simulink model "scExampleAutomotiveElectricalSystemAnalysis"  (R2024a)
settings: Solver=VariableStepAuto  StartTime=0.0  StopTime=10.0  RelTol=1e-3
(part 2 of 2)

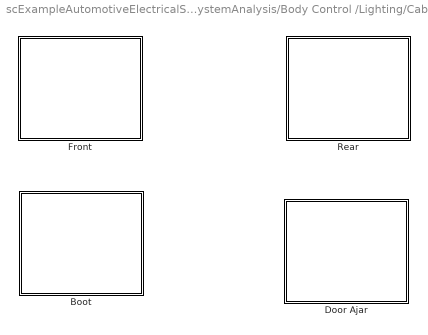
== system scExampleAutomotiveElectricalSystemAnalysis/Body Control /Lighting/Cabin lights ==
  Boot : Subsystem
      settings: PortSchema="{\"entries\":[{\"content\":{\"headerSize\":26,\"margin\":15,\"minimumSpacing\":25,\"sides\":[{\"content\":{\"connectorIds\":[]},\"type\":\"ConnectorPlacement.EquallySpacedRectSide\",\"uuid\":\"3d65bb45-329f-4bcb-b2ca-42a1dcaed35c\"},{\"content\":{\"connectorIds\":[],\"side\":\"RIGHT\"},\"type\":\"ConnectorPlacement.EquallySpacedRectSide\",\"uuid\":\"712ce926-4e36-4f57-ab01-804e3d1e4b50\"},{\"content\":{\"connectorIds\":[],\"side\":\"TOP\"},\"type\":\"ConnectorPlacement.EquallySpacedRectSide\",\"uuid\":\"e185dea3-2ee8-4adb-8a1b-2283728bdd8a\"}]},\"type\":\"ConnectorPlacement.EquallySpacedConnector\",\"uuid\":\"16f1484a-02ca-4d23-9e19-71fd982c775e\"}],\"packageUris\":[\"http:\\/\\/schema.mathworks.com\\/mf0\\/Connector\\/19700101\"],\"version\":\"1.0\"}"
  Door Ajar : Subsystem
      settings: PortSchema="{\"entries\":[{\"content\":{\"headerSize\":26,\"margin\":15,\"minimumSpacing\":25,\"sides\":[{\"content\":{\"connectorIds\":[]},\"type\":\"ConnectorPlacement.EquallySpacedRectSide\",\"uuid\":\"3d65bb45-329f-4bcb-b2ca-42a1dcaed35c\"},{\"content\":{\"connectorIds\":[],\"side\":\"RIGHT\"},\"type\":\"ConnectorPlacement.EquallySpacedRectSide\",\"uuid\":\"712ce926-4e36-4f57-ab01-804e3d1e4b50\"},{\"content\":{\"connectorIds\":[],\"side\":\"TOP\"},\"type\":\"ConnectorPlacement.EquallySpacedRectSide\",\"uuid\":\"e185dea3-2ee8-4adb-8a1b-2283728bdd8a\"}]},\"type\":\"ConnectorPlacement.EquallySpacedConnector\",\"uuid\":\"16f1484a-02ca-4d23-9e19-71fd982c775e\"}],\"packageUris\":[\"http:\\/\\/schema.mathworks.com\\/mf0\\/Connector\\/19700101\"],\"version\":\"1.0\"}"
  Front : Subsystem
      settings: PortSchema="{\"entries\":[{\"content\":{\"headerSize\":26,\"margin\":15,\"minimumSpacing\":25,\"sides\":[{\"content\":{\"connectorIds\":[]},\"type\":\"ConnectorPlacement.EquallySpacedRectSide\",\"uuid\":\"3d65bb45-329f-4bcb-b2ca-42a1dcaed35c\"},{\"content\":{\"connectorIds\":[],\"side\":\"RIGHT\"},\"type\":\"ConnectorPlacement.EquallySpacedRectSide\",\"uuid\":\"712ce926-4e36-4f57-ab01-804e3d1e4b50\"},{\"content\":{\"connectorIds\":[],\"side\":\"TOP\"},\"type\":\"ConnectorPlacement.EquallySpacedRectSide\",\"uuid\":\"e185dea3-2ee8-4adb-8a1b-2283728bdd8a\"}]},\"type\":\"ConnectorPlacement.EquallySpacedConnector\",\"uuid\":\"16f1484a-02ca-4d23-9e19-71fd982c775e\"}],\"packageUris\":[\"http:\\/\\/schema.mathworks.com\\/mf0\\/Connector\\/19700101\"],\"version\":\"1.0\"}"
  Rear : Subsystem
      settings: PortSchema="{\"entries\":[{\"content\":{\"headerSize\":26,\"margin\":15,\"minimumSpacing\":25,\"sides\":[{\"content\":{\"connectorIds\":[]},\"type\":\"ConnectorPlacement.EquallySpacedRectSide\",\"uuid\":\"3d65bb45-329f-4bcb-b2ca-42a1dcaed35c\"},{\"content\":{\"connectorIds\":[],\"side\":\"RIGHT\"},\"type\":\"ConnectorPlacement.EquallySpacedRectSide\",\"uuid\":\"712ce926-4e36-4f57-ab01-804e3d1e4b50\"},{\"content\":{\"connectorIds\":[],\"side\":\"TOP\"},\"type\":\"ConnectorPlacement.EquallySpacedRectSide\",\"uuid\":\"e185dea3-2ee8-4adb-8a1b-2283728bdd8a\"}]},\"type\":\"ConnectorPlacement.EquallySpacedConnector\",\"uuid\":\"16f1484a-02ca-4d23-9e19-71fd982c775e\"}],\"packageUris\":[\"http:\\/\\/schema.mathworks.com\\/mf0\\/Connector\\/19700101\"],\"version\":\"1.0\"}"

== system scExampleAutomotiveElectricalSystemAnalysis/Body Control /Lighting/Fog lamps ==
  Front : Subsystem
      settings: PortSchema="{\"entries\":[{\"content\":{\"headerSize\":26,\"margin\":15,\"minimumSpacing\":25,\"sides\":[{\"content\":{\"connectorIds\":[]},\"type\":\"ConnectorPlacement.EquallySpacedRectSide\",\"uuid\":\"3d65bb45-329f-4bcb-b2ca-42a1dcaed35c\"},{\"content\":{\"connectorIds\":[],\"side\":\"RIGHT\"},\"type\":\"ConnectorPlacement.EquallySpacedRectSide\",\"uuid\":\"712ce926-4e36-4f57-ab01-804e3d1e4b50\"},{\"content\":{\"connectorIds\":[],\"side\":\"TOP\"},\"type\":\"ConnectorPlacement.EquallySpacedRectSide\",\"uuid\":\"e185dea3-2ee8-4adb-8a1b-2283728bdd8a\"}]},\"type\":\"ConnectorPlacement.EquallySpacedConnector\",\"uuid\":\"16f1484a-02ca-4d23-9e19-71fd982c775e\"}],\"packageUris\":[\"http:\\/\\/schema.mathworks.com\\/mf0\\/Connector\\/19700101\"],\"version\":\"1.0\"}"
  Rear : Subsystem
      settings: PortSchema="{\"entries\":[{\"content\":{\"headerSize\":26,\"margin\":15,\"minimumSpacing\":25,\"sides\":[{\"content\":{\"connectorIds\":[]},\"type\":\"ConnectorPlacement.EquallySpacedRectSide\",\"uuid\":\"3d65bb45-329f-4bcb-b2ca-42a1dcaed35c\"},{\"content\":{\"connectorIds\":[],\"side\":\"RIGHT\"},\"type\":\"ConnectorPlacement.EquallySpacedRectSide\",\"uuid\":\"712ce926-4e36-4f57-ab01-804e3d1e4b50\"},{\"content\":{\"connectorIds\":[],\"side\":\"TOP\"},\"type\":\"ConnectorPlacement.EquallySpacedRectSide\",\"uuid\":\"e185dea3-2ee8-4adb-8a1b-2283728bdd8a\"}]},\"type\":\"ConnectorPlacement.EquallySpacedConnector\",\"uuid\":\"16f1484a-02ca-4d23-9e19-71fd982c775e\"}],\"packageUris\":[\"http:\\/\\/schema.mathworks.com\\/mf0\\/Connector\\/19700101\"],\"version\":\"1.0\"}"

== system scExampleAutomotiveElectricalSystemAnalysis/Body Control /Lighting/Hazard lamps ==

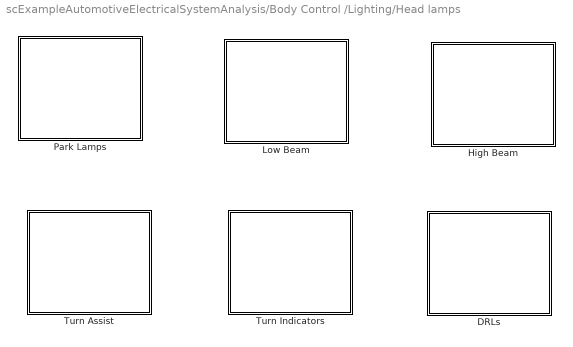
== system scExampleAutomotiveElectricalSystemAnalysis/Body Control /Lighting/Head lamps ==
  DRLs : Subsystem
      settings: PortSchema="{\"entries\":[{\"content\":{\"headerSize\":26,\"margin\":15,\"minimumSpacing\":25,\"sides\":[{\"content\":{\"connectorIds\":[]},\"type\":\"ConnectorPlacement.EquallySpacedRectSide\",\"uuid\":\"3d65bb45-329f-4bcb-b2ca-42a1dcaed35c\"},{\"content\":{\"connectorIds\":[],\"side\":\"RIGHT\"},\"type\":\"ConnectorPlacement.EquallySpacedRectSide\",\"uuid\":\"712ce926-4e36-4f57-ab01-804e3d1e4b50\"},{\"content\":{\"connectorIds\":[],\"side\":\"TOP\"},\"type\":\"ConnectorPlacement.EquallySpacedRectSide\",\"uuid\":\"e185dea3-2ee8-4adb-8a1b-2283728bdd8a\"}]},\"type\":\"ConnectorPlacement.EquallySpacedConnector\",\"uuid\":\"16f1484a-02ca-4d23-9e19-71fd982c775e\"}],\"packageUris\":[\"http:\\/\\/schema.mathworks.com\\/mf0\\/Connector\\/19700101\"],\"version\":\"1.0\"}"
  High Beam : Subsystem
      settings: PortSchema="{\"entries\":[{\"content\":{\"headerSize\":26,\"margin\":15,\"minimumSpacing\":25,\"sides\":[{\"content\":{\"connectorIds\":[]},\"type\":\"ConnectorPlacement.EquallySpacedRectSide\",\"uuid\":\"3d65bb45-329f-4bcb-b2ca-42a1dcaed35c\"},{\"content\":{\"connectorIds\":[],\"side\":\"RIGHT\"},\"type\":\"ConnectorPlacement.EquallySpacedRectSide\",\"uuid\":\"712ce926-4e36-4f57-ab01-804e3d1e4b50\"},{\"content\":{\"connectorIds\":[],\"side\":\"TOP\"},\"type\":\"ConnectorPlacement.EquallySpacedRectSide\",\"uuid\":\"e185dea3-2ee8-4adb-8a1b-2283728bdd8a\"}]},\"type\":\"ConnectorPlacement.EquallySpacedConnector\",\"uuid\":\"16f1484a-02ca-4d23-9e19-71fd982c775e\"}],\"packageUris\":[\"http:\\/\\/schema.mathworks.com\\/mf0\\/Connector\\/19700101\"],\"version\":\"1.0\"}"
  Low Beam : Subsystem
      settings: PortSchema="{\"entries\":[{\"content\":{\"headerSize\":26,\"margin\":15,\"minimumSpacing\":25,\"sides\":[{\"content\":{\"connectorIds\":[]},\"type\":\"ConnectorPlacement.EquallySpacedRectSide\",\"uuid\":\"3d65bb45-329f-4bcb-b2ca-42a1dcaed35c\"},{\"content\":{\"connectorIds\":[],\"side\":\"RIGHT\"},\"type\":\"ConnectorPlacement.EquallySpacedRectSide\",\"uuid\":\"712ce926-4e36-4f57-ab01-804e3d1e4b50\"},{\"content\":{\"connectorIds\":[],\"side\":\"TOP\"},\"type\":\"ConnectorPlacement.EquallySpacedRectSide\",\"uuid\":\"e185dea3-2ee8-4adb-8a1b-2283728bdd8a\"}]},\"type\":\"ConnectorPlacement.EquallySpacedConnector\",\"uuid\":\"16f1484a-02ca-4d23-9e19-71fd982c775e\"}],\"packageUris\":[\"http:\\/\\/schema.mathworks.com\\/mf0\\/Connector\\/19700101\"],\"version\":\"1.0\"}"
  Park Lamps : Subsystem
      settings: PortSchema="{\"entries\":[{\"content\":{\"headerSize\":26,\"margin\":15,\"minimumSpacing\":25,\"sides\":[{\"content\":{\"connectorIds\":[]},\"type\":\"ConnectorPlacement.EquallySpacedRectSide\",\"uuid\":\"3d65bb45-329f-4bcb-b2ca-42a1dcaed35c\"},{\"content\":{\"connectorIds\":[],\"side\":\"RIGHT\"},\"type\":\"ConnectorPlacement.EquallySpacedRectSide\",\"uuid\":\"712ce926-4e36-4f57-ab01-804e3d1e4b50\"},{\"content\":{\"connectorIds\":[],\"side\":\"TOP\"},\"type\":\"ConnectorPlacement.EquallySpacedRectSide\",\"uuid\":\"e185dea3-2ee8-4adb-8a1b-2283728bdd8a\"}]},\"type\":\"ConnectorPlacement.EquallySpacedConnector\",\"uuid\":\"16f1484a-02ca-4d23-9e19-71fd982c775e\"}],\"packageUris\":[\"http:\\/\\/schema.mathworks.com\\/mf0\\/Connector\\/19700101\"],\"version\":\"1.0\"}"
  Turn Assist : Subsystem
      settings: PortSchema="{\"entries\":[{\"content\":{\"headerSize\":26,\"margin\":15,\"minimumSpacing\":25,\"sides\":[{\"content\":{\"connectorIds\":[]},\"type\":\"ConnectorPlacement.EquallySpacedRectSide\",\"uuid\":\"3d65bb45-329f-4bcb-b2ca-42a1dcaed35c\"},{\"content\":{\"connectorIds\":[],\"side\":\"RIGHT\"},\"type\":\"ConnectorPlacement.EquallySpacedRectSide\",\"uuid\":\"712ce926-4e36-4f57-ab01-804e3d1e4b50\"},{\"content\":{\"connectorIds\":[],\"side\":\"TOP\"},\"type\":\"ConnectorPlacement.EquallySpacedRectSide\",\"uuid\":\"e185dea3-2ee8-4adb-8a1b-2283728bdd8a\"}]},\"type\":\"ConnectorPlacement.EquallySpacedConnector\",\"uuid\":\"16f1484a-02ca-4d23-9e19-71fd982c775e\"}],\"packageUris\":[\"http:\\/\\/schema.mathworks.com\\/mf0\\/Connector\\/19700101\"],\"version\":\"1.0\"}"
  Turn Indicators : Subsystem
      settings: PortSchema="{\"entries\":[{\"content\":{\"headerSize\":26,\"margin\":15,\"minimumSpacing\":25,\"sides\":[{\"content\":{\"connectorIds\":[]},\"type\":\"ConnectorPlacement.EquallySpacedRectSide\",\"uuid\":\"3d65bb45-329f-4bcb-b2ca-42a1dcaed35c\"},{\"content\":{\"connectorIds\":[],\"side\":\"RIGHT\"},\"type\":\"ConnectorPlacement.EquallySpacedRectSide\",\"uuid\":\"712ce926-4e36-4f57-ab01-804e3d1e4b50\"},{\"content\":{\"connectorIds\":[],\"side\":\"TOP\"},\"type\":\"ConnectorPlacement.EquallySpacedRectSide\",\"uuid\":\"e185dea3-2ee8-4adb-8a1b-2283728bdd8a\"}]},\"type\":\"ConnectorPlacement.EquallySpacedConnector\",\"uuid\":\"16f1484a-02ca-4d23-9e19-71fd982c775e\"}],\"packageUris\":[\"http:\\/\\/schema.mathworks.com\\/mf0\\/Connector\\/19700101\"],\"version\":\"1.0\"}"

== system scExampleAutomotiveElectricalSystemAnalysis/Body Control /Lighting/Tail lamps ==
  Brake lights : Subsystem
      settings: PortSchema="{\"entries\":[{\"content\":{\"headerSize\":26,\"margin\":15,\"minimumSpacing\":25,\"sides\":[{\"content\":{\"connectorIds\":[]},\"type\":\"ConnectorPlacement.EquallySpacedRectSide\",\"uuid\":\"3d65bb45-329f-4bcb-b2ca-42a1dcaed35c\"},{\"content\":{\"connectorIds\":[],\"side\":\"RIGHT\"},\"type\":\"ConnectorPlacement.EquallySpacedRectSide\",\"uuid\":\"712ce926-4e36-4f57-ab01-804e3d1e4b50\"},{\"content\":{\"connectorIds\":[],\"side\":\"TOP\"},\"type\":\"ConnectorPlacement.EquallySpacedRectSide\",\"uuid\":\"e185dea3-2ee8-4adb-8a1b-2283728bdd8a\"}]},\"type\":\"ConnectorPlacement.EquallySpacedConnector\",\"uuid\":\"16f1484a-02ca-4d23-9e19-71fd982c775e\"}],\"packageUris\":[\"http:\\/\\/schema.mathworks.com\\/mf0\\/Connector\\/19700101\"],\"version\":\"1.0\"}"
  Reversing lamps : Subsystem
      settings: PortSchema="{\"entries\":[{\"content\":{\"headerSize\":26,\"margin\":15,\"minimumSpacing\":25,\"sides\":[{\"content\":{\"connectorIds\":[]},\"type\":\"ConnectorPlacement.EquallySpacedRectSide\",\"uuid\":\"3d65bb45-329f-4bcb-b2ca-42a1dcaed35c\"},{\"content\":{\"connectorIds\":[],\"side\":\"RIGHT\"},\"type\":\"ConnectorPlacement.EquallySpacedRectSide\",\"uuid\":\"712ce926-4e36-4f57-ab01-804e3d1e4b50\"},{\"content\":{\"connectorIds\":[],\"side\":\"TOP\"},\"type\":\"ConnectorPlacement.EquallySpacedRectSide\",\"uuid\":\"e185dea3-2ee8-4adb-8a1b-2283728bdd8a\"}]},\"type\":\"ConnectorPlacement.EquallySpacedConnector\",\"uuid\":\"16f1484a-02ca-4d23-9e19-71fd982c775e\"}],\"packageUris\":[\"http:\\/\\/schema.mathworks.com\\/mf0\\/Connector\\/19700101\"],\"version\":\"1.0\"}"
  Tail lights : Subsystem
      settings: PortSchema="{\"entries\":[{\"content\":{\"headerSize\":26,\"margin\":15,\"minimumSpacing\":25,\"sides\":[{\"content\":{\"connectorIds\":[]},\"type\":\"ConnectorPlacement.EquallySpacedRectSide\",\"uuid\":\"3d65bb45-329f-4bcb-b2ca-42a1dcaed35c\"},{\"content\":{\"connectorIds\":[],\"side\":\"RIGHT\"},\"type\":\"ConnectorPlacement.EquallySpacedRectSide\",\"uuid\":\"712ce926-4e36-4f57-ab01-804e3d1e4b50\"},{\"content\":{\"connectorIds\":[],\"side\":\"TOP\"},\"type\":\"ConnectorPlacement.EquallySpacedRectSide\",\"uuid\":\"e185dea3-2ee8-4adb-8a1b-2283728bdd8a\"}]},\"type\":\"ConnectorPlacement.EquallySpacedConnector\",\"uuid\":\"16f1484a-02ca-4d23-9e19-71fd982c775e\"}],\"packageUris\":[\"http:\\/\\/schema.mathworks.com\\/mf0\\/Connector\\/19700101\"],\"version\":\"1.0\"}"

== system scExampleAutomotiveElectricalSystemAnalysis/Body Control /Wipers & Washers/Head lamps ==

== system scExampleAutomotiveElectricalSystemAnalysis/Body Control /Wipers & Washers/Tail gate ==

== system scExampleAutomotiveElectricalSystemAnalysis/Body Control /Wipers & Washers/Wind Screen ==

== system scExampleAutomotiveElectricalSystemAnalysis/Comfort/HVAC/Blower ==

== system scExampleAutomotiveElectricalSystemAnalysis/Comfort/HVAC/Climate Control ==

== system scExampleAutomotiveElectricalSystemAnalysis/Comfort/HVAC/Radiator Fan ==

== system scExampleAutomotiveElectricalSystemAnalysis/Comfort/Infotainment/Amplifier ==

== system scExampleAutomotiveElectricalSystemAnalysis/Comfort/Infotainment/Headrest Displays ==

== system scExampleAutomotiveElectricalSystemAnalysis/Comfort/Infotainment/Navigation System ==

== system scExampleAutomotiveElectricalSystemAnalysis/Comfort/Infotainment/Radio ==

== system scExampleAutomotiveElectricalSystemAnalysis/Body Control /Lighting/Cabin lights/Boot ==

== system scExampleAutomotiveElectricalSystemAnalysis/Body Control /Lighting/Cabin lights/Door Ajar ==

== system scExampleAutomotiveElectricalSystemAnalysis/Body Control /Lighting/Cabin lights/Front ==

== system scExampleAutomotiveElectricalSystemAnalysis/Body Control /Lighting/Cabin lights/Rear ==

== system scExampleAutomotiveElectricalSystemAnalysis/Body Control /Lighting/Fog lamps/Front ==

== system scExampleAutomotiveElectricalSystemAnalysis/Body Control /Lighting/Fog lamps/Rear ==

== system scExampleAutomotiveElectricalSystemAnalysis/Body Control /Lighting/Head lamps/DRLs ==

== system scExampleAutomotiveElectricalSystemAnalysis/Body Control /Lighting/Head lamps/High Beam ==

== system scExampleAutomotiveElectricalSystemAnalysis/Body Control /Lighting/Head lamps/Low Beam ==

== system scExampleAutomotiveElectricalSystemAnalysis/Body Control /Lighting/Head lamps/Park Lamps ==

== system scExampleAutomotiveElectricalSystemAnalysis/Body Control /Lighting/Head lamps/Turn Assist ==

== system scExampleAutomotiveElectricalSystemAnalysis/Body Control /Lighting/Head lamps/Turn Indicators ==

== system scExampleAutomotiveElectricalSystemAnalysis/Body Control /Lighting/Tail lamps/Brake lights ==

== system scExampleAutomotiveElectricalSystemAnalysis/Body Control /Lighting/Tail lamps/Reversing lamps ==

== system scExampleAutomotiveElectricalSystemAnalysis/Body Control /Lighting/Tail lamps/Tail lights ==
